simulink model "TTS_4motor_simplify_PMSM_ver2"  (R2020b)
settings: Solver=VariableStepAuto  StartTime=0.0  StopTime=0.8  RelTol=1e-3
InitFcn:
  | C = 0.015 % 中间直流电路的电容
  | f = 50 %频率
  | Rn = 0.01 % 整流部分电阻
  | Ln = 0.0012; % 整流电路部分电感
  | Udcref = 800*sqrt(2)
  | Un = 350
  | 
  | noiseDense = 1e-4 % 速度传感器故障噪声
  | 
  | w = 2*pi*f
  | 
  | np=2;
  | Tloadmax  = 50 % 最大负载
  | Tloadstart = 0.35 % 负载添加时间
  | Tdiscrete = 2e-6 % 离散时间
  | t_precharge = 0.15 % 整流预充电
  | Tpwm = 5e-4 % 逆变 PWM 周期
  | Ts = 1e-4
  | sample_time = Tdiscrete; % scope 采样时间
  | 
  | %基础参数
  | Rs_ref=0.43
  | Lm_ref=0.0006931
  | J_ref=0.1
  | Rflux_ref = 0.175
  | 
  | 
  | %电机 1 参数
  | Rflux1=0.9618*Rflux_ref
  | Rs1=0.9874*Rs_ref
  | Lm1=0.9747*Lm_ref
  | J1=0.9645*J_ref
  | 
  | 
  | %电机 2 参数
  | Rflux2=1.0145*Rflux_ref
  | Rs2=0.9810*Rs_ref
  | Lm2=0.9963*Lm_ref
  | J2=1.0415*J_ref
  | 
  | 
  | %电机 3 参数
  | Rflux3=1.0317*Rflux_ref
  | Rs3=0.9948*Rs_ref
  | Lm3=0.9914*Lm_ref
  | J3=1.0269*J_ref
  | 
  | 
  | %电机 4 参数
  | Rflux4=1.0481*Rflux_ref
  | Rs4=0.9914*Rs_ref
  | Lm4=0.9938*Lm_ref
  | J4=0.9873*J_ref
  | 
  | 
  | 
  | % 故障设置参数
  | % 速度传感器
  | tE1w = 10.3
  | 
  | ... (+21 lines)
undefined symbols (not defined in the file): m1_pA
libraries: powerlib x23, simulink x11, pid_lib x1, eeSinusoidalMeasurementV2 x1
(part 2 of 2)

== system TTS_4motor_simplify_PMSM_ver2/Subsystem/SVPWM1/find section1/not neg ==
  In1 : Inport
  Constant2 : Constant  Value=0
  Relational Operator : RelationalOperator  OutDataTypeStr=boolean  RndMeth=Simplest
  Out1 : Outport
  wires:
  In1/1 -> Relational Operator/1
  Relational Operator/1 -> Out1/1
  Constant2/1 -> Relational Operator/2

== system TTS_4motor_simplify_PMSM_ver2/Subsystem/SVPWM1/find section1/not neg1 ==
  In1 : Inport
  Constant2 : Constant  Value=0
  Relational Operator : RelationalOperator  OutDataTypeStr=boolean  RndMeth=Simplest
  Out1 : Outport
  wires:
  Constant2/1 -> Relational Operator/2
  Relational Operator/1 -> Out1/1
  In1/1 -> Relational Operator/1

== system TTS_4motor_simplify_PMSM_ver2/Subsystem1/SVPWM1/find section1/>=0? ==
  In1 : Inport
  Constant2 : Constant  Value=0
  Relational Operator : RelationalOperator  OutDataTypeStr=boolean  RndMeth=Simplest
  Out1 : Outport
  wires:
  In1/1 -> Relational Operator/1
  Relational Operator/1 -> Out1/1
  Constant2/1 -> Relational Operator/2

== system TTS_4motor_simplify_PMSM_ver2/Subsystem1/SVPWM1/find section1/not neg ==
  In1 : Inport
  Constant2 : Constant  Value=0
  Relational Operator : RelationalOperator  OutDataTypeStr=boolean  RndMeth=Simplest
  Out1 : Outport
  wires:
  Constant2/1 -> Relational Operator/2
  Relational Operator/1 -> Out1/1
  In1/1 -> Relational Operator/1

== system TTS_4motor_simplify_PMSM_ver2/Subsystem1/SVPWM1/find section1/not neg1 ==
  In1 : Inport
  Constant2 : Constant  Value=0
  Relational Operator : RelationalOperator  OutDataTypeStr=boolean  RndMeth=Simplest
  Out1 : Outport
  wires:
  In1/1 -> Relational Operator/1
  Relational Operator/1 -> Out1/1
  Constant2/1 -> Relational Operator/2

== system TTS_4motor_simplify_PMSM_ver2/Subsystem2/SVPWM1/find section1/>=0? ==
  In1 : Inport
  Constant2 : Constant  Value=0
  Relational Operator : RelationalOperator  OutDataTypeStr=boolean  RndMeth=Simplest
  Out1 : Outport
  wires:
  Constant2/1 -> Relational Operator/2
  Relational Operator/1 -> Out1/1
  In1/1 -> Relational Operator/1

== system TTS_4motor_simplify_PMSM_ver2/Subsystem2/SVPWM1/find section1/not neg ==
  In1 : Inport
  Constant2 : Constant  Value=0
  Relational Operator : RelationalOperator  OutDataTypeStr=boolean  RndMeth=Simplest
  Out1 : Outport
  wires:
  In1/1 -> Relational Operator/1
  Relational Operator/1 -> Out1/1
  Constant2/1 -> Relational Operator/2

== system TTS_4motor_simplify_PMSM_ver2/Subsystem2/SVPWM1/find section1/not neg1 ==
  In1 : Inport
  Constant2 : Constant  Value=0
  Relational Operator : RelationalOperator  OutDataTypeStr=boolean  RndMeth=Simplest
  Out1 : Outport
  wires:
  Constant2/1 -> Relational Operator/2
  Relational Operator/1 -> Out1/1
  In1/1 -> Relational Operator/1

== system TTS_4motor_simplify_PMSM_ver2/Subsystem3/SVPWM1/find section1/>=0? ==
  In1 : Inport
  Constant2 : Constant  Value=0
  Relational Operator : RelationalOperator  OutDataTypeStr=boolean  RndMeth=Simplest
  Out1 : Outport
  wires:
  In1/1 -> Relational Operator/1
  Relational Operator/1 -> Out1/1
  Constant2/1 -> Relational Operator/2

== system TTS_4motor_simplify_PMSM_ver2/Subsystem3/SVPWM1/find section1/not neg ==
  In1 : Inport
  Constant2 : Constant  Value=0
  Relational Operator : RelationalOperator  OutDataTypeStr=boolean  RndMeth=Simplest
  Out1 : Outport
  wires:
  Constant2/1 -> Relational Operator/2
  Relational Operator/1 -> Out1/1
  In1/1 -> Relational Operator/1

== system TTS_4motor_simplify_PMSM_ver2/Subsystem3/SVPWM1/find section1/not neg1 ==
  In1 : Inport
  Constant2 : Constant  Value=0
  Relational Operator : RelationalOperator  OutDataTypeStr=boolean  RndMeth=Simplest
  Out1 : Outport
  wires:
  In1/1 -> Relational Operator/1
  Relational Operator/1 -> Out1/1
  Constant2/1 -> Relational Operator/2

== matlab function TTS_4motor_simplify_PMSM_ver2/Subsystem1/SVPWM1/MATLAB Function ==
  data: Udcref input; ua_ output; ua input; ub input; ub_ output
function [ua_, ub_] = fcn(Udcref, ua, ub)

I = sqrt(ua*ua + ub*ub);

if(I == 0)
    I = 1;
end

ua_ = ua / I * Udcref/sqrt(3);
ub_ = ub / I * Udcref/sqrt(3);

== matlab function TTS_4motor_simplify_PMSM_ver2/Subsystem1/SVPWM1/MATLAB Function10 ==
  data: Ta input; gA output; Tb input; Tpwm input; section input; t input; gAN output; gB output; gBN output; gC output; gCN output
function [gA,gAN, gB, gBN, gC, gCN]  = fcn(Ta, Tb, Tpwm, section, t)

gA = (1==1);
gB = (1==1);
gC = (1==1);

T0 = Tpwm - Ta - Tb;

% 七段式 SPWM，扇区 1~6，对应6个扇区

if(mod(section, 2) == 1 ) % 1、3、5扇区
    t1 = T0/4;
    t2 = t1 + Ta / 2;
    t3 = t2 + Tb / 2;
    t4 = t3 + T0 / 2;
    t5 = t4 + Tb / 2;
    t6 = t5 + Ta / 2;
    
    if(section == 1)
        gA = (t >=t1 && t <=t6);
        gB = (t >=t2 && t <= t5);
        gC = (t >=t3 && t <= t4);
    elseif(section == 3)
        gB = (t >=t1 && t <=t6);
        gC = (t >=t2 && t <= t5);
        gA = (t >=t3 && t <= t4);
    else
        gC = (t >=t1 && t <=t6);
        gA = (t >=t2 && t <= t5);
        gB = (t >=t3 && t <= t4);
    end
else
    t1 = T0/4;
    t2 = t1 + Tb / 2;
    t3 = t2 + Ta / 2;
    t4 = t3 + T0 / 2;
    t5 = t4 + Ta / 2;
    t6 = t5 + Tb / 2;
    
    if(section == 2)
        gB = (t >=t1 && t <=t6);
        gA = (t >=t2 && t <= t5);
        gC = (t >=t3 && t <= t4);
    elseif(section == 4)
        gC = (t >=t1 && t <=t6);
        gB = (t >=t2 && t <= t5);
        gA = (t >=t3 && t <= t4);
    else
        gA = (t >=t1 && t <=t6);
        gC = (t >=t2 && t <= t5);
        gB = (t >=t3 && t <= t4);        
    end
    
end


gAN = ~gA;
gBN = ~gB;
gCN = ~gC;
% g = [gA, 1-gA, gB, 1-gB, gC, 1-gC];

== matlab function TTS_4motor_simplify_PMSM_ver2/Subsystem1/SVPWM1/MATLAB Function3 ==
  data: Udc input; T0 output; Ualpha input; Ubeta input; Ts input; sec input; T1 output; T2 output

function [T0, T1, T2] = fcn( Udc, Ualpha, Ubeta,  Ts, sec)
co = cos((sec-1)*pi/3);
si = sin((sec-1)*pi/3);

Ualpha_ = Ualpha*co + Ubeta*si;
Ubeta_ = -Ualpha*si + Ubeta*co;


T2 = sqrt(3)*Ubeta_/Udc*Ts;
T1 = ( 3*Ualpha_ - sqrt(3)* Ubeta_)/2/Udc*Ts;
T0 = Ts - T1 - T2;

== matlab function TTS_4motor_simplify_PMSM_ver2/Subsystem/SVPWM1/MATLAB Function3 ==
  data: Udc input; T0 output; Ualpha input; Ubeta input; Ts input; sec input; T1 output; T2 output

function [T0, T1, T2] = fcn( Udc, Ualpha, Ubeta,  Ts, sec)
co = cos((sec-1)*pi/3);
si = sin((sec-1)*pi/3);

Ualpha_ = Ualpha*co + Ubeta*si;
Ubeta_ = -Ualpha*si + Ubeta*co;


T2 = sqrt(3)*Ubeta_/Udc*Ts;
T1 = ( 3*Ualpha_ - sqrt(3)* Ubeta_)/2/Udc*Ts;
T0 = Ts - T1 - T2;

== matlab function TTS_4motor_simplify_PMSM_ver2/Subsystem1/SVPWM1/find section1/get section ==
  data: u input; y output
function y = fcn(u)
switch u
    case 5
        y = 1;
    case 7
        y = 2; 
    case 6
        y = 3;
    case 2
        y = 4;
    case 0
        y = 5;
    case 1
        y = 6;
    otherwise
        y = 0;
end

== matlab function TTS_4motor_simplify_PMSM_ver2/Subsystem2/MATLAB Function2 ==
  data: A input; alpha output; B input; C input; beta output
function [alpha, beta] = fcn(A, B, C)
k = 2/ 3;
alpha = k * (A - 0.5*B - 0.5*C);
beta = k * sqrt(3) / 2 * (B - C);

== matlab function TTS_4motor_simplify_PMSM_ver2/Subsystem2/MATLAB Function4 ==
  data: Im output; Ialpha input; Ibeta input; theta input; It output
function [Im, It] = fcn(Ialpha, Ibeta, theta)

Im = Ialpha * cos(theta) + Ibeta * sin(theta);
It = -Ialpha * sin(theta) + Ibeta * cos(theta);

== matlab function TTS_4motor_simplify_PMSM_ver2/Subsystem1/MATLAB Function2 ==
  data: A input; alpha output; B input; C input; beta output
function [alpha, beta] = fcn(A, B, C)
k = 2/ 3;
alpha = k * (A - 0.5*B - 0.5*C);
beta = k * sqrt(3) / 2 * (B - C);

== matlab function TTS_4motor_simplify_PMSM_ver2/Subsystem/SVPWM1/find section1/get section ==
  data: u input; y output
function y = fcn(u)
switch u
    case 5
        y = 1;
    case 7
        y = 2; 
    case 6
        y = 3;
    case 2
        y = 4;
    case 0
        y = 5;
    case 1
        y = 6;
    otherwise
        y = 0;
end

== matlab function TTS_4motor_simplify_PMSM_ver2/Subsystem2/MATLAB Function6 ==
  data: alpha output; m input; t input; theta input; beta output
function [alpha, beta] = fcn(m, t, theta)

alpha = cos(theta) * m - sin(theta) * t;
beta = sin(theta) * m + cos(theta) * t;

== matlab function TTS_4motor_simplify_PMSM_ver2/Subsystem2/SVPWM1/MATLAB Function ==
  data: Udcref input; ua_ output; ua input; ub input; ub_ output
function [ua_, ub_] = fcn(Udcref, ua, ub)

I = sqrt(ua*ua + ub*ub);

if(I == 0)
    I = 1;
end

ua_ = ua / I * Udcref/sqrt(3);
ub_ = ub / I * Udcref/sqrt(3);

== matlab function TTS_4motor_simplify_PMSM_ver2/Subsystem2/SVPWM1/MATLAB Function10 ==
  data: Ta input; gA output; Tb input; Tpwm input; section input; t input; gAN output; gB output; gBN output; gC output; gCN output
function [gA,gAN, gB, gBN, gC, gCN]  = fcn(Ta, Tb, Tpwm, section, t)

gA = (1==1);
gB = (1==1);
gC = (1==1);

T0 = Tpwm - Ta - Tb;

% 七段式 SPWM，扇区 1~6，对应6个扇区

if(mod(section, 2) == 1 ) % 1、3、5扇区
    t1 = T0/4;
    t2 = t1 + Ta / 2;
    t3 = t2 + Tb / 2;
    t4 = t3 + T0 / 2;
    t5 = t4 + Tb / 2;
    t6 = t5 + Ta / 2;
    
    if(section == 1)
        gA = (t >=t1 && t <=t6);
        gB = (t >=t2 && t <= t5);
        gC = (t >=t3 && t <= t4);
    elseif(section == 3)
        gB = (t >=t1 && t <=t6);
        gC = (t >=t2 && t <= t5);
        gA = (t >=t3 && t <= t4);
    else
        gC = (t >=t1 && t <=t6);
        gA = (t >=t2 && t <= t5);
        gB = (t >=t3 && t <= t4);
    end
else
    t1 = T0/4;
    t2 = t1 + Tb / 2;
    t3 = t2 + Ta / 2;
    t4 = t3 + T0 / 2;
    t5 = t4 + Ta / 2;
    t6 = t5 + Tb / 2;
    
    if(section == 2)
        gB = (t >=t1 && t <=t6);
        gA = (t >=t2 && t <= t5);
        gC = (t >=t3 && t <= t4);
    elseif(section == 4)
        gC = (t >=t1 && t <=t6);
        gB = (t >=t2 && t <= t5);
        gA = (t >=t3 && t <= t4);
    else
        gA = (t >=t1 && t <=t6);
        gC = (t >=t2 && t <= t5);
        gB = (t >=t3 && t <= t4);        
    end
    
end


gAN = ~gA;
gBN = ~gB;
gCN = ~gC;
% g = [gA, 1-gA, gB, 1-gB, gC, 1-gC];

== matlab function TTS_4motor_simplify_PMSM_ver2/Subsystem2/SVPWM1/MATLAB Function3 ==
  data: Udc input; T0 output; Ualpha input; Ubeta input; Ts input; sec input; T1 output; T2 output

function [T0, T1, T2] = fcn( Udc, Ualpha, Ubeta,  Ts, sec)
co = cos((sec-1)*pi/3);
si = sin((sec-1)*pi/3);

Ualpha_ = Ualpha*co + Ubeta*si;
Ubeta_ = -Ualpha*si + Ubeta*co;


T2 = sqrt(3)*Ubeta_/Udc*Ts;
T1 = ( 3*Ualpha_ - sqrt(3)* Ubeta_)/2/Udc*Ts;
T0 = Ts - T1 - T2;

== matlab function TTS_4motor_simplify_PMSM_ver2/Subsystem2/SVPWM1/find section1/get section ==
  data: u input; y output
function y = fcn(u)
switch u
    case 5
        y = 1;
    case 7
        y = 2; 
    case 6
        y = 3;
    case 2
        y = 4;
    case 0
        y = 5;
    case 1
        y = 6;
    otherwise
        y = 0;
end

== matlab function TTS_4motor_simplify_PMSM_ver2/Subsystem3/MATLAB Function2 ==
  data: A input; alpha output; B input; C input; beta output
function [alpha, beta] = fcn(A, B, C)
k = 2/ 3;
alpha = k * (A - 0.5*B - 0.5*C);
beta = k * sqrt(3) / 2 * (B - C);

== matlab function TTS_4motor_simplify_PMSM_ver2/Subsystem3/MATLAB Function4 ==
  data: Im output; Ialpha input; Ibeta input; theta input; It output
function [Im, It] = fcn(Ialpha, Ibeta, theta)

Im = Ialpha * cos(theta) + Ibeta * sin(theta);
It = -Ialpha * sin(theta) + Ibeta * cos(theta);

== matlab function TTS_4motor_simplify_PMSM_ver2/Subsystem3/MATLAB Function6 ==
  data: alpha output; m input; t input; theta input; beta output
function [alpha, beta] = fcn(m, t, theta)

alpha = cos(theta) * m - sin(theta) * t;
beta = sin(theta) * m + cos(theta) * t;

== matlab function TTS_4motor_simplify_PMSM_ver2/Subsystem3/SVPWM1/MATLAB Function ==
  data: Udcref input; ua_ output; ua input; ub input; ub_ output
function [ua_, ub_] = fcn(Udcref, ua, ub)

I = sqrt(ua*ua + ub*ub);

if(I == 0)
    I = 1;
end

ua_ = ua / I * Udcref/sqrt(3);
ub_ = ub / I * Udcref/sqrt(3);

== matlab function TTS_4motor_simplify_PMSM_ver2/Subsystem1/MATLAB Function4 ==
  data: Im output; Ialpha input; Ibeta input; theta input; It output
function [Im, It] = fcn(Ialpha, Ibeta, theta)

Im = Ialpha * cos(theta) + Ibeta * sin(theta);
It = -Ialpha * sin(theta) + Ibeta * cos(theta);

== matlab function TTS_4motor_simplify_PMSM_ver2/Subsystem3/SVPWM1/MATLAB Function10 ==
  data: Ta input; gA output; Tb input; Tpwm input; section input; t input; gAN output; gB output; gBN output; gC output; gCN output
function [gA,gAN, gB, gBN, gC, gCN]  = fcn(Ta, Tb, Tpwm, section, t)

gA = (1==1);
gB = (1==1);
gC = (1==1);

T0 = Tpwm - Ta - Tb;

% 七段式 SPWM，扇区 1~6，对应6个扇区

if(mod(section, 2) == 1 ) % 1、3、5扇区
    t1 = T0/4;
    t2 = t1 + Ta / 2;
    t3 = t2 + Tb / 2;
    t4 = t3 + T0 / 2;
    t5 = t4 + Tb / 2;
    t6 = t5 + Ta / 2;
    
    if(section == 1)
        gA = (t >=t1 && t <=t6);
        gB = (t >=t2 && t <= t5);
        gC = (t >=t3 && t <= t4);
    elseif(section == 3)
        gB = (t >=t1 && t <=t6);
        gC = (t >=t2 && t <= t5);
        gA = (t >=t3 && t <= t4);
    else
        gC = (t >=t1 && t <=t6);
        gA = (t >=t2 && t <= t5);
        gB = (t >=t3 && t <= t4);
    end
else
    t1 = T0/4;
    t2 = t1 + Tb / 2;
    t3 = t2 + Ta / 2;
    t4 = t3 + T0 / 2;
    t5 = t4 + Ta / 2;
    t6 = t5 + Tb / 2;
    
    if(section == 2)
        gB = (t >=t1 && t <=t6);
        gA = (t >=t2 && t <= t5);
        gC = (t >=t3 && t <= t4);
    elseif(section == 4)
        gC = (t >=t1 && t <=t6);
        gB = (t >=t2 && t <= t5);
        gA = (t >=t3 && t <= t4);
    else
        gA = (t >=t1 && t <=t6);
        gC = (t >=t2 && t <= t5);
        gB = (t >=t3 && t <= t4);        
    end
    
end


gAN = ~gA;
gBN = ~gB;
gCN = ~gC;
% g = [gA, 1-gA, gB, 1-gB, gC, 1-gC];

== matlab function TTS_4motor_simplify_PMSM_ver2/Subsystem3/SVPWM1/MATLAB Function3 ==
  data: Udc input; T0 output; Ualpha input; Ubeta input; Ts input; sec input; T1 output; T2 output

function [T0, T1, T2] = fcn( Udc, Ualpha, Ubeta,  Ts, sec)
co = cos((sec-1)*pi/3);
si = sin((sec-1)*pi/3);

Ualpha_ = Ualpha*co + Ubeta*si;
Ubeta_ = -Ualpha*si + Ubeta*co;


T2 = sqrt(3)*Ubeta_/Udc*Ts;
T1 = ( 3*Ualpha_ - sqrt(3)* Ubeta_)/2/Udc*Ts;
T0 = Ts - T1 - T2;

== matlab function TTS_4motor_simplify_PMSM_ver2/Subsystem3/SVPWM1/find section1/get section ==
  data: u input; y output
function y = fcn(u)
switch u
    case 5
        y = 1;
    case 7
        y = 2; 
    case 6
        y = 3;
    case 2
        y = 4;
    case 0
        y = 5;
    case 1
        y = 6;
    otherwise
        y = 0;
end

== matlab function TTS_4motor_simplify_PMSM_ver2/MATLAB Function1 ==
  data: t input; lower input; upper input; Tload input; y output
function y = fcn( t, lower, upper,Tload)

if (t <= upper && t >= lower) 
    y = Tload;
elseif(t >= upper)
    y = Tload;
else
    y = 0;
end

== matlab function TTS_4motor_simplify_PMSM_ver2/MATLAB Function ==
  data: n_ref input; nr1 input; nr1_ output; nr2_ output; nr3_ output; nr2 input; nr3 input; nr4 input; nr4_ output
function [nr1_, nr2_, nr3_, nr4_] = fcn(n_ref, nr1, nr2, nr3, nr4)

% K1 = 0;
% K2 = 0;
% K3 = 0;
% K4 = 0;

% K1 = 0.50;
% K2 = 0.30;
% K3 = 0.20;
% K4 = 0.15;

K1 = 50;
K2 = 30;
K3 = 20;
K4 = 15;

nr1_  = n_ref - nr1 - K1*(nr1 - nr2) - K3*(nr1 - nr3) - K4*(nr1 - nr4);
nr2_  = n_ref - nr2 - K1*(nr2 - nr1) - K2*(nr2 - nr3) - K3*(nr2 - nr4);
nr3_  = n_ref - nr3 - K3*(nr3 - nr1) - K2*(nr3 - nr2) - K1*(nr3 - nr4);
nr4_  = n_ref - nr4 - K4*(nr4 - nr1) - K3*(nr4 - nr2) - K1*(nr4 - nr3);

% nr1_  = nr1 + 0.3*(nr1 - nr2) + 0.3*(nr1 - nr3) + 0.3*(nr1 - nr4);
% nr2_  = nr2 + 0.3*(nr2 - nr1) + 0.3*(nr2 - nr3) + 0.3*(nr2 - nr4);
% nr3_  = nr3 + 0.3*(nr3 - nr1) + 0.3*(nr3 - nr2) + 0.3*(nr3 - nr4);
% nr4_  = nr4 + 0.3*(nr4 - nr1) + 0.3*(nr4 - nr2) + 0.3*(nr4 - nr3);

== matlab function TTS_4motor_simplify_PMSM_ver2/Subsystem/MATLAB Function2 ==
  data: A input; alpha output; B input; C input; beta output
function [alpha, beta] = fcn(A, B, C)
k = 2/ 3;
alpha = k * (A - 0.5*B - 0.5*C);
beta = k * sqrt(3) / 2 * (B - C);

== matlab function TTS_4motor_simplify_PMSM_ver2/Subsystem1/MATLAB Function6 ==
  data: alpha output; m input; t input; theta input; beta output
function [alpha, beta] = fcn(m, t, theta)

alpha = cos(theta) * m - sin(theta) * t;
beta = sin(theta) * m + cos(theta) * t;

== matlab function TTS_4motor_simplify_PMSM_ver2/Subsystem/MATLAB Function4 ==
  data: Im output; Ialpha input; Ibeta input; theta input; It output
function [Im, It] = fcn(Ialpha, Ibeta, theta)

Im = Ialpha * cos(theta) + Ibeta * sin(theta);
It = -Ialpha * sin(theta) + Ibeta * cos(theta);

== matlab function TTS_4motor_simplify_PMSM_ver2/Subsystem/MATLAB Function6 ==
  data: alpha output; m input; t input; theta input; beta output
function [alpha, beta] = fcn(m, t, theta)

alpha = cos(theta) * m - sin(theta) * t;
beta = sin(theta) * m + cos(theta) * t;

== matlab function TTS_4motor_simplify_PMSM_ver2/Subsystem/SVPWM1/MATLAB Function10 ==
  data: Ta input; gA output; Tb input; Tpwm input; section input; t input; gAN output; gB output; gBN output; gC output; gCN output
function [gA,gAN, gB, gBN, gC, gCN]  = fcn(Ta, Tb, Tpwm, section, t)

gA = (1==1);
gB = (1==1);
gC = (1==1);

T0 = Tpwm - Ta - Tb;

% 七段式 SPWM，扇区 1~6，对应6个扇区

if(mod(section, 2) == 1 ) % 1、3、5扇区
    t1 = T0/4;
    t2 = t1 + Ta / 2;
    t3 = t2 + Tb / 2;
    t4 = t3 + T0 / 2;
    t5 = t4 + Tb / 2;
    t6 = t5 + Ta / 2;
    
    if(section == 1)
        gA = (t >=t1 && t <=t6);
        gB = (t >=t2 && t <= t5);
        gC = (t >=t3 && t <= t4);
    elseif(section == 3)
        gB = (t >=t1 && t <=t6);
        gC = (t >=t2 && t <= t5);
        gA = (t >=t3 && t <= t4);
    else
        gC = (t >=t1 && t <=t6);
        gA = (t >=t2 && t <= t5);
        gB = (t >=t3 && t <= t4);
    end
else
    t1 = T0/4;
    t2 = t1 + Tb / 2;
    t3 = t2 + Ta / 2;
    t4 = t3 + T0 / 2;
    t5 = t4 + Ta / 2;
    t6 = t5 + Tb / 2;
    
    if(section == 2)
        gB = (t >=t1 && t <=t6);
        gA = (t >=t2 && t <= t5);
        gC = (t >=t3 && t <= t4);
    elseif(section == 4)
        gC = (t >=t1 && t <=t6);
        gB = (t >=t2 && t <= t5);
        gA = (t >=t3 && t <= t4);
    else
        gA = (t >=t1 && t <=t6);
        gC = (t >=t2 && t <= t5);
        gB = (t >=t3 && t <= t4);        
    end
    
end


gAN = ~gA;
gBN = ~gB;
gCN = ~gC;
% g = [gA, 1-gA, gB, 1-gB, gC, 1-gC];

== matlab function TTS_4motor_simplify_PMSM_ver2/Subsystem/SVPWM1/避免幅值过大 ==
  data: Udcref input; ua_ output; ua input; ub input; ub_ output
function [ua_, ub_] = fcn(Udcref, ua, ub)

I = sqrt(ua*ua + ub*ub);

if(I == 0)
    I = 1;
end

ua_ = ua / I * Udcref/sqrt(3);
ub_ = ub / I * Udcref/sqrt(3);
